simulink model "coord_alpha_test"  (R2014b)
settings: Solver=ode45  StartTime=0.0  StopTime=10.0  RelTol=1e-3
libraries: QuaternionLib x5
settings Model: Creator=5909  LastModifiedBy=5909

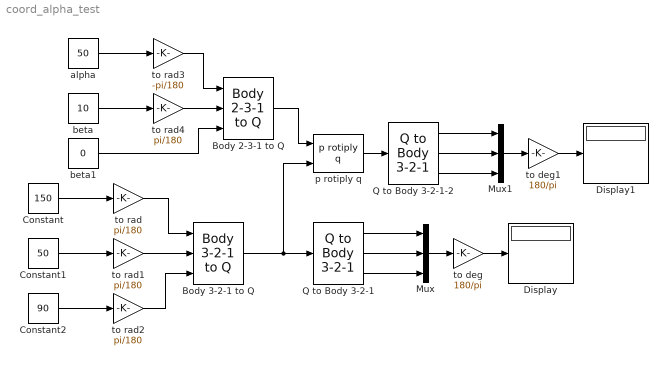
== system coord_alpha_test ==
  Body 2-3-1 to Q : QuaternionLib/Body 2-3-1 to Q
  Body 3-2-1 to Q : QuaternionLib/Body 3-2-1 to Q
  Constant : Constant  Value=150
  Constant1 : Constant  Value=50
  Constant2 : Constant  Value=90
  Display : Display
  Display1 : Display
  Mux : Mux  Inputs=3
  Mux1 : Mux  Inputs=3
  Q to Body 3-2-1 : QuaternionLib/Q to Body 3-2-1
  "Q to Body 3-2-1-2 " : QuaternionLib/Q to Body 3-2-1
  alpha : Constant  Value=50
  beta : Constant  Value=10
  beta1 : Constant  Value=0
  p rotiply q : QuaternionLib/p rotiply q
  to deg : Gain  Gain=180/pi
  to deg1 : Gain  Gain=180/pi
  to rad{,1..2,4} (4 alike) : Gain  Gain=pi/180
  to rad3 : Gain  Gain=-pi/180
  wires:
  Body 3-2-1 to Q/1 -> p rotiply q/2, Q to Body 3-2-1/1
  to rad/1 -> Body 3-2-1 to Q/1
  Constant/1 -> to rad/1
  to rad1/1 -> Body 3-2-1 to Q/2
  Constant1/1 -> to rad1/1
  to rad2/1 -> Body 3-2-1 to Q/3
  Constant2/1 -> to rad2/1
  Q to Body 3-2-1/2 -> Mux/2
  Q to Body 3-2-1/1 -> Mux/1
  Q to Body 3-2-1/3 -> Mux/3
  Mux/1 -> to deg/1
  to deg/1 -> Display/1
  Body 2-3-1 to Q/1 -> p rotiply q/1
  alpha/1 -> to rad3/1
  beta/1 -> to rad4/1
  to rad3/1 -> Body 2-3-1 to Q/1
  to rad4/1 -> Body 2-3-1 to Q/2
  beta1/1 -> Body 2-3-1 to Q/3
  p rotiply q/1 -> "Q to Body 3-2-1-2 "/1
  "Q to Body 3-2-1-2 "/2 -> Mux1/2
  "Q to Body 3-2-1-2 "/1 -> Mux1/1
  "Q to Body 3-2-1-2 "/3 -> Mux1/3
  Mux1/1 -> to deg1/1
  to deg1/1 -> Display1/1
